simulink library "Simulation_lib"  (R2023b)
settings: Solver=VariableStepAuto  StartTime=0.0  StopTime=10.0  RelTol=1e-3
undefined symbols (not defined in the file): X, Y, Z
libraries: sm_lib x48, $bdroot x18, nesl_utility x16, fl_lib x15, ee_lib x3, simulink_extras x1
(part 1 of 3)
settings Model: Creator=FIRSTMentor  LastModifiedBy=FIRSTMentor

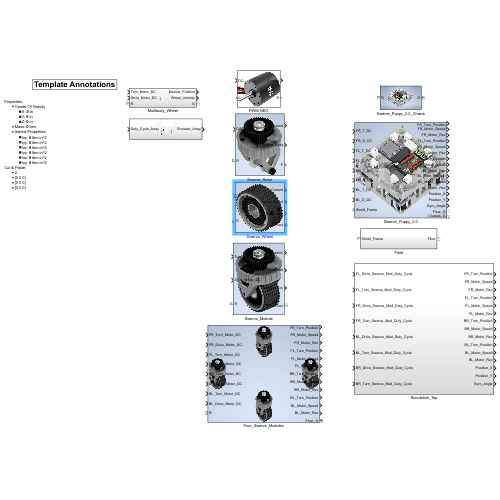
[thumbnail: Simulink's stored preview of the top-level diagram]
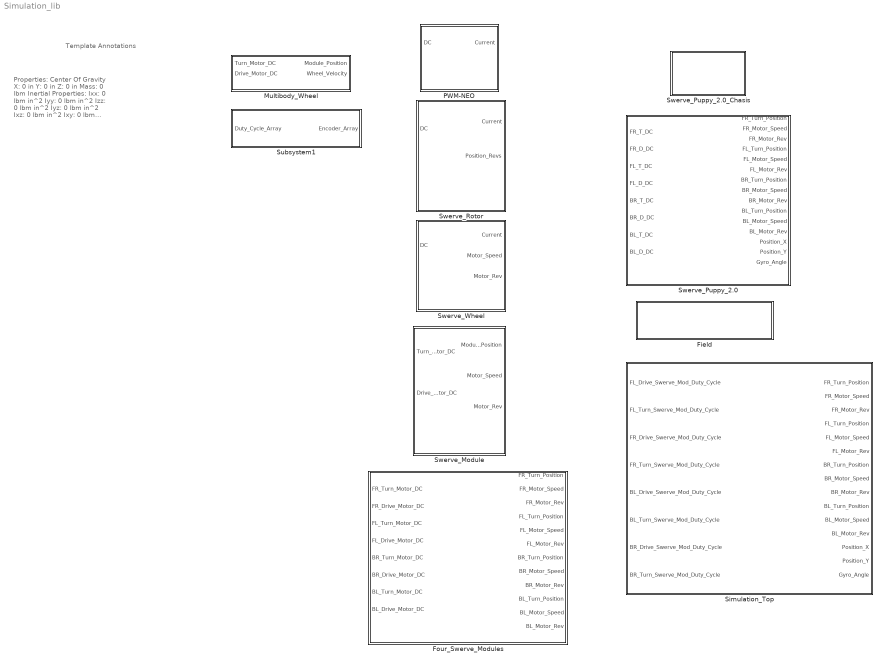
== system Simulation_lib ==
  note: Properties:
      | Center Of Gravity
      | X: 0 in
      | Y: 0 in
      | Z: 0 in
      | Mass: 0 lbm
      | Inertial Properties:
      | Ixx: 0 lbm in^2
      | Iyy: 0 lbm in^2
      | Izz: 0 lbm in^2
      | Iyz: 0 lbm in^2
      | Ixz: 0 lbm in^2
      | Ixy: 0 lbm in^2
      | Cut & Paste:
      | 0
      | [0 0 0]
      | [0 0 0]
      | [0 0 0]
  note: Template Annotations
  Field : Subsystem
  Four_Swerve_Modules : Subsystem  mask{FR_Transform=[0 0 0], FL_Transform=[0 0 0], BR_Transform=[0 0 0], BL_Transform=[0 0 0]}
      mask prompts: FR_Transform "Front Right Module Transform"; FL_Transform "Front Left Module Transform"; BR_Transform "Back Right Module Transform"; BL_Transform "Back Right Module Transform"
      mask DialogControl Instructions Prompt: Only enter the X and Y of transforms, Z should always be zero.
      mask Display: image('Four_Swerve_Modules_Icon.png'); % Use "Edit Image" on toolstrip to change.
  Multibody_Wheel : Subsystem
  PWM-NEO : Subsystem
      mask Display: image('NEO_Icon.png'); % Use "Edit Image" on toolstrip to change.
  Simulation_Top : Subsystem
  Subsystem1 : Subsystem
  Swerve_Module : Subsystem
      mask Display: image('Swerve_Wheel_Module_Icon.png'); % Use "Edit Image" on toolstrip to change.
  Swerve_Puppy_2.0 : Subsystem
      mask Display: image('Swerve_Puppy_2.0_Icon.png'); % Use "Edit Image" on toolstrip to change.
  Swerve_Puppy_2.0_Chasis : Subsystem
      mask Display: image('Swerve_Puppy_2.0_Chassis_Icon.png'); % Use "Edit Image" on toolstrip to change.
  Swerve_Rotor : Subsystem
      mask Display: image('Swerve_Rotor_Icon.png'); % Use "Edit Image" on toolstrip to change.
  Swerve_Wheel : Subsystem
      mask Display: image('Swerve_Wheel_Icon.png'); % Use "Edit Image" on toolstrip to change.

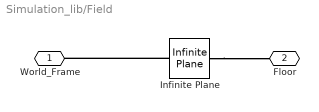
== system Simulation_lib/Field ==
  Infinite Plane : sm_lib/Curves and Surfaces/Infinite Plane  GraphicType=Rectangle  GraphicPlaneWidth=10  GraphicPlaneWidthUnits=m  GraphicPlaneHeight=10  GraphicPlaneHeightUnits=m  GraphicVisPropType=SimpleVisualProperties  GraphicDiffuseColor=[1 0.4118 0.1608]  GraphicOpacity=0.25  GraphicSpecularColor=[0.5 0.5 0.5 1.0]  GraphicAmbientColor=[0.15 0.15 0.15 1.0]  GraphicEmissiveColor=[0.0 0.0 0.0 1.0]  GraphicShininess=75
  World_Frame : PMIOPort  Side=Left
  Floor : PMIOPort  Port=2  Side=Right
  connections:
  Infinite Plane/RConn1 -- Floor/RConn1
  Infinite Plane/LConn1 -- World_Frame/RConn1

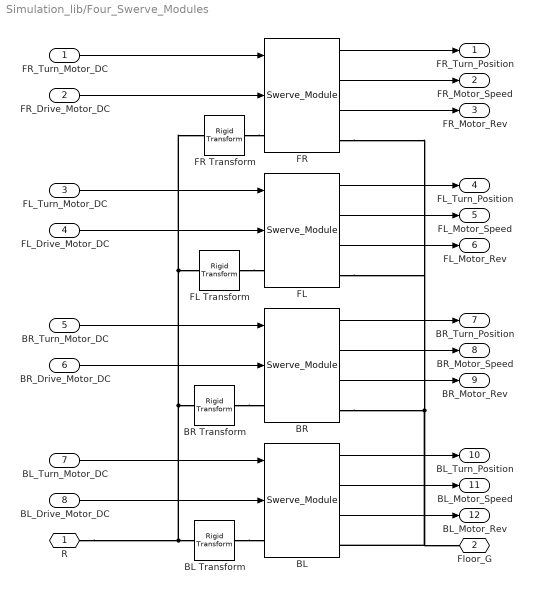
== system Simulation_lib/Four_Swerve_Modules ==
  FR_Turn_Motor_DC : Inport
  FR_Drive_Motor_DC : Inport  Port=2
  FL_Turn_Motor_DC : Inport  Port=3
  FL_Drive_Motor_DC : Inport  Port=4
  BR_Turn_Motor_DC : Inport  Port=5
  BR_Drive_Motor_DC : Inport  Port=6
  BL_Turn_Motor_DC : Inport  Port=7
  BL_Drive_Motor_DC : Inport  Port=8
  BL : $bdroot/Swerve_Module  SystemSampleTime=-1  VariantActivationTime=update diagram  AllowFlexibleInterface=on  Latency=0  AutoFrameSizeCalculation=off
  BL Transform : sm_lib/Frames and Transforms/Rigid Transform  TranslationMethod=Cartesian  TranslationStandardOffset=0  TranslationStandardOffsetUnits=m  TranslationStandardAxis=+Z  TranslationCartesianOffset=BL_Transform  TranslationCartesianOffsetUnits=in  TranslationROffset=0  TranslationROffsetUnits=m  TranslationZOffset=0  TranslationZOffsetUnits=m  TranslationThetaOffset=0  TranslationThetaOffsetUnits=deg  RotationMethod=None  RotationAngleUnits=deg  RotationStandardAxis=+Z  RotationAngle=0.0  RotationArbitraryAxis=[0 0 1]  FollAlignAxisA=+X  BaseAlignAxisA=+Y  FollAlignAxisB=+Y  BaseAlignAxisB=+Z  RotationSequenceAxes=FollowerAxes  RotationSequence=XYX  RotationSequenceAngles=[0 0 0]  RotationSequenceAnglesUnits=deg  RotationMatrix=[1 0 0; 0 1 0; 0 0 1]  Quaternion=[1 0 0 0]
  BR : $bdroot/Swerve_Module  SystemSampleTime=-1  VariantActivationTime=update diagram  AllowFlexibleInterface=on  Latency=0  AutoFrameSizeCalculation=off
  BR Transform : sm_lib/Frames and Transforms/Rigid Transform  TranslationMethod=Cartesian  TranslationStandardOffset=0  TranslationStandardOffsetUnits=m  TranslationStandardAxis=+Z  TranslationCartesianOffset=BR_Transform  TranslationCartesianOffsetUnits=in  TranslationROffset=0  TranslationROffsetUnits=m  TranslationZOffset=0  TranslationZOffsetUnits=m  TranslationThetaOffset=0  TranslationThetaOffsetUnits=deg  RotationMethod=None  RotationAngleUnits=deg  RotationStandardAxis=+Z  RotationAngle=0.0  RotationArbitraryAxis=[0 0 1]  FollAlignAxisA=+X  BaseAlignAxisA=+Y  FollAlignAxisB=+Y  BaseAlignAxisB=+Z  RotationSequenceAxes=FollowerAxes  RotationSequence=XYX  RotationSequenceAngles=[0 0 0]  RotationSequenceAnglesUnits=deg  RotationMatrix=[1 0 0; 0 1 0; 0 0 1]  Quaternion=[1 0 0 0]
  FL : $bdroot/Swerve_Module  SystemSampleTime=-1  VariantActivationTime=update diagram  AllowFlexibleInterface=on  Latency=0  AutoFrameSizeCalculation=off
  FL Transform : sm_lib/Frames and Transforms/Rigid Transform  TranslationMethod=Cartesian  TranslationStandardOffset=0  TranslationStandardOffsetUnits=m  TranslationStandardAxis=+Z  TranslationCartesianOffset=FL_Transform  TranslationCartesianOffsetUnits=in  TranslationROffset=0  TranslationROffsetUnits=m  TranslationZOffset=0  TranslationZOffsetUnits=m  TranslationThetaOffset=0  TranslationThetaOffsetUnits=deg  RotationMethod=None  RotationAngleUnits=deg  RotationStandardAxis=+Z  RotationAngle=0.0  RotationArbitraryAxis=[0 0 1]  FollAlignAxisA=+X  BaseAlignAxisA=+Y  FollAlignAxisB=+Y  BaseAlignAxisB=+Z  RotationSequenceAxes=FollowerAxes  RotationSequence=XYX  RotationSequenceAngles=[0 0 0]  RotationSequenceAnglesUnits=deg  RotationMatrix=[1 0 0; 0 1 0; 0 0 1]  Quaternion=[1 0 0 0]
  FR : $bdroot/Swerve_Module  SystemSampleTime=-1  VariantActivationTime=update diagram  AllowFlexibleInterface=on  Latency=0  AutoFrameSizeCalculation=off
  FR Transform : sm_lib/Frames and Transforms/Rigid Transform  TranslationMethod=Cartesian  TranslationStandardOffset=0  TranslationStandardOffsetUnits=m  TranslationStandardAxis=+Z  TranslationCartesianOffset=FR_Transform  TranslationCartesianOffsetUnits=in  TranslationROffset=0  TranslationROffsetUnits=m  TranslationZOffset=0  TranslationZOffsetUnits=m  TranslationThetaOffset=0  TranslationThetaOffsetUnits=deg  RotationMethod=None  RotationAngleUnits=deg  RotationStandardAxis=+Z  RotationAngle=0.0  RotationArbitraryAxis=[0 0 1]  FollAlignAxisA=+X  BaseAlignAxisA=+Y  FollAlignAxisB=+Y  BaseAlignAxisB=+Z  RotationSequenceAxes=FollowerAxes  RotationSequence=XYX  RotationSequenceAngles=[0 0 0]  RotationSequenceAnglesUnits=deg  RotationMatrix=[1 0 0; 0 1 0; 0 0 1]  Quaternion=[1 0 0 0]
  R : PMIOPort  Side=Left
  Floor_G : PMIOPort  Port=2  Side=Right
  FR_Turn_Position : Outport
  FR_Motor_Speed : Outport  Port=2
  FR_Motor_Rev : Outport  Port=3  Unit=rev
  FL_Turn_Position : Outport  Port=4
  FL_Motor_Speed : Outport  Port=5
  FL_Motor_Rev : Outport  Port=6  Unit=rev
  BR_Turn_Position : Outport  Port=7
  BR_Motor_Speed : Outport  Port=8
  BR_Motor_Rev : Outport  Port=9  Unit=rev
  BL_Turn_Position : Outport  Port=10
  BL_Motor_Speed : Outport  Port=11
  BL_Motor_Rev : Outport  Port=12  Unit=rev
  wires:
  FR_Turn_Motor_DC/1 -> FR/1
  FR_Drive_Motor_DC/1 -> FR/2
  FL_Drive_Motor_DC/1 -> FL/2
  FL_Turn_Motor_DC/1 -> FL/1
  BR_Turn_Motor_DC/1 -> BR/1
  BR_Drive_Motor_DC/1 -> BR/2
  BL_Turn_Motor_DC/1 -> BL/1
  BL_Drive_Motor_DC/1 -> BL/2
  BL/2 -> BL_Motor_Speed/1
  BL/1 -> BL_Turn_Position/1
  BR/1 -> BR_Turn_Position/1
  BR/2 -> BR_Motor_Speed/1
  FL/1 -> FL_Turn_Position/1
  FL/2 -> FL_Motor_Speed/1
  FR/1 -> FR_Turn_Position/1
  FR/2 -> FR_Motor_Speed/1
  FR/3 -> FR_Motor_Rev/1
  FL/3 -> FL_Motor_Rev/1
  BR/3 -> BR_Motor_Rev/1
  BL/3 -> BL_Motor_Rev/1
  connections:
  R/RConn1 -- FL Transform/LConn1 -- FR Transform/LConn1 -- BR Transform/LConn1 -- BL Transform/LConn1
  BL/RConn1 -- Floor_G/RConn1 -- FR/RConn1 -- FL/RConn1 -- BR/RConn1
  FR Transform/RConn1 -- FR/LConn1
  FL Transform/RConn1 -- FL/LConn1
  BR Transform/RConn1 -- BR/LConn1
  BL Transform/RConn1 -- BL/LConn1

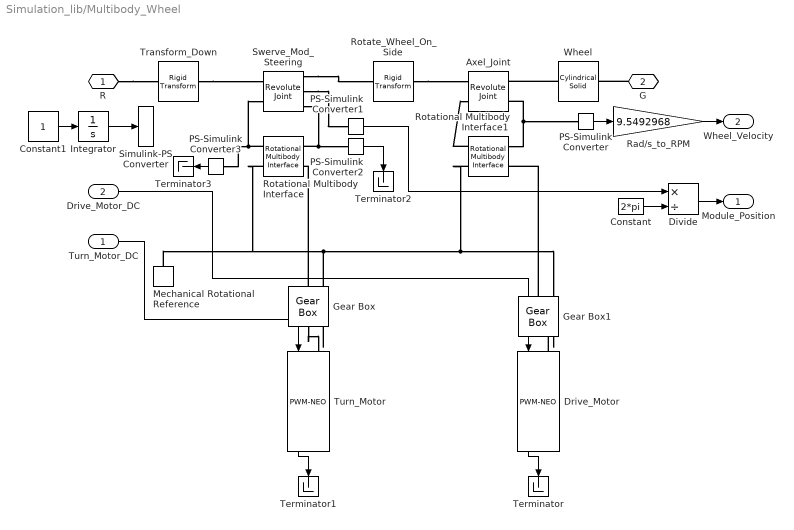
== system Simulation_lib/Multibody_Wheel ==
  Turn_Motor_DC : Inport
  Drive_Motor_DC : Inport  Port=2
  Axel_Joint : sm_lib/Joints/Revolute Joint  JointMode=Normal  SenseConstraintForce=off  SenseConstraintForceX=off  SenseConstraintForceY=off  SenseConstraintForceZ=off  SenseConstraintTorque=off  SenseConstraintTorqueX=off  SenseConstraintTorqueY=off  SenseConstraintTorqueZ=off  SenseTotalForce=off  SenseTotalForceX=off  SenseTotalForceY=off  SenseTotalForceZ=off  SenseTotalTorque=off  SenseTotalTorqueX=off  SenseTotalTorqueY=off  SenseTotalTorqueZ=off  CompositeWrenchDir=FollowerOnBase  CompositeWrenchFrame=BaseFrame  EquilibriumPosition=0  EquilibriumPositionUnits=deg  SpringStiffness=0  SpringStiffnessUnits=N*m/deg  DampingCoefficient=0  DampingCoefficientUnits=N*m/(deg/s)  TorqueActuationMode=InputTorque  MotionActuationMode=ComputedMotion  SensePosition=off  SenseVelocity=on  SenseAcceleration=off  SenseTorqueForce=off  SenseLowerLimitTorqueForce=off  SenseUpperLimitTorqueForce=off  LowerLimitSpecify=off  LowerLimitBound=-90  LowerLimitBoundUnits=deg  LowerLimitStiffness=1e4  LowerLimitStiffnessUnits=N*m/deg  LowerLimitDamping=10  LowerLimitDampingUnits=N*m/(deg/s)  LowerLimitTransitionRegionWidth=0.1  LowerLimitTransitionRegionWidthUnits=deg  UpperLimitSpecify=off  UpperLimitBound=90  UpperLimitBoundUnits=deg  UpperLimitStiffness=1e4  UpperLimitStiffnessUnits=N*m/deg  UpperLimitDamping=10  UpperLimitDampingUnits=N*m/(deg/s)  UpperLimitTransitionRegionWidth=0.1  UpperLimitTransitionRegionWidthUnits=deg  PositionTargetSpecify=off  PositionTargetPriority=High  PositionTargetValue=0  PositionTargetValueUnits=deg  VelocityTargetSpecify=off  VelocityTargetPriority=High  VelocityTargetValue=0  VelocityTargetValueUnits=deg/s
  Constant : Constant  Value=2*pi
  Constant1 : Constant
  Divide : Product  Inputs=*/
  Drive_Motor : $bdroot/PWM-NEO  SystemSampleTime=-1  VariantActivationTime=update diagram  AllowFlexibleInterface=on  Latency=0  AutoFrameSizeCalculation=off
  Gear Box : fl_lib/Mechanical/Mechanisms/Gear Box  ratio=150/7  t_in_specify=off  t_in_priority=None  t_in=0 N*m  t_in_nominal_specify=off  t_in_nominal_unit=N*m  t_in_nominal_value=1  t_out_specify=off  t_out_priority=None  t_out=0 N*m  t_out_nominal_specify=off  t_out_nominal_unit=N*m  t_out_nominal_value=1
  Gear Box1 : fl_lib/Mechanical/Mechanisms/Gear Box  ratio=8.14  t_in_specify=off  t_in_priority=None  t_in=0 N*m  t_in_nominal_specify=off  t_in_nominal_unit=N*m  t_in_nominal_value=1  t_out_specify=off  t_out_priority=None  t_out=0 N*m  t_out_nominal_specify=off  t_out_nominal_unit=N*m  t_out_nominal_value=1
  Integrator : Integrator
  Mechanical Rotational Reference : fl_lib/Mechanical/Rotational Elements/Mechanical Rotational Reference
  PS-Simulink Converter{,1..3} (4 alike) : nesl_utility/PS-Simulink Converter  PhysicalDomain=network_engine_domain  SubClassName=ps_output  LeftPortType=input  RightPortType=output  PseudoPeriodic=off  Frequencies=[]  VectorFormat=inherit  Unit=inherit  AffineConversion=off
  Rad/s_to_RPM : Gain  Gain=9.5492968
  Rotate_Wheel_On_Side : sm_lib/Frames and Transforms/Rigid Transform  TranslationMethod=None  TranslationStandardOffset=0  TranslationStandardOffsetUnits=m  TranslationStandardAxis=+Z  TranslationCartesianOffset=[0 0 0]  TranslationCartesianOffsetUnits=m  TranslationROffset=0  TranslationROffsetUnits=m  TranslationZOffset=0  TranslationZOffsetUnits=m  TranslationThetaOffset=0  TranslationThetaOffsetUnits=deg  RotationMethod=StandardAxis  RotationAngleUnits=deg  RotationStandardAxis=+X  RotationAngle=90  RotationArbitraryAxis=[0 0 1]  FollAlignAxisA=+X  BaseAlignAxisA=+Y  FollAlignAxisB=+Y  BaseAlignAxisB=+Z  RotationSequenceAxes=FollowerAxes  RotationSequence=XYX  RotationSequenceAngles=[0 0 0]  RotationSequenceAnglesUnits=deg  RotationMatrix=[1 0 0; 0 1 0; 0 0 1]  Quaternion=[1 0 0 0]
  Rotational Multibody Interface : fl_lib/Mechanical/Multibody Interfaces/Rotational Multibody Interface
  Rotational Multibody Interface1 : fl_lib/Mechanical/Multibody Interfaces/Rotational Multibody Interface
  Simulink-PS Converter : nesl_utility/Simulink-PS Converter  PhysicalDomain=network_engine_domain  SubClassName=ps_input  LeftPortType=input  RightPortType=output  PseudoPeriodic=off  Frequencies=[]  NoiseDistribution=none  NoiseParameters=[]  Unit=1  AffineConversion=on  FilteringAndDerivatives=filter  SimscapeFilterOrder=2  InputFilterTimeConstant=0.001  UdotUserProvided=2
  Swerve_Mod_Steering : sm_lib/Joints/Revolute Joint  JointMode=Normal  SenseConstraintForce=off  SenseConstraintForceX=off  SenseConstraintForceY=off  SenseConstraintForceZ=off  SenseConstraintTorque=off  SenseConstraintTorqueX=off  SenseConstraintTorqueY=off  SenseConstraintTorqueZ=off  SenseTotalForce=off  SenseTotalForceX=off  SenseTotalForceY=off  SenseTotalForceZ=off  SenseTotalTorque=off  SenseTotalTorqueX=off  SenseTotalTorqueY=off  SenseTotalTorqueZ=off  CompositeWrenchDir=FollowerOnBase  CompositeWrenchFrame=BaseFrame  EquilibriumPosition=0  EquilibriumPositionUnits=deg  SpringStiffness=0  SpringStiffnessUnits=N*m/deg  DampingCoefficient=0  DampingCoefficientUnits=N*m/(deg/s)  TorqueActuationMode=InputTorque  MotionActuationMode=ComputedMotion  SensePosition=on  SenseVelocity=on  SenseAcceleration=off  SenseTorqueForce=off  SenseLowerLimitTorqueForce=off  SenseUpperLimitTorqueForce=off  LowerLimitSpecify=off  LowerLimitBound=-90  LowerLimitBoundUnits=deg  LowerLimitStiffness=1e4  LowerLimitStiffnessUnits=N*m/deg  LowerLimitDamping=10  LowerLimitDampingUnits=N*m/(deg/s)  LowerLimitTransitionRegionWidth=0.1  LowerLimitTransitionRegionWidthUnits=deg  UpperLimitSpecify=off  UpperLimitBound=90  UpperLimitBoundUnits=deg  UpperLimitStiffness=1e4  UpperLimitStiffnessUnits=N*m/deg  UpperLimitDamping=10  UpperLimitDampingUnits=N*m/(deg/s)  UpperLimitTransitionRegionWidth=0.1  UpperLimitTransitionRegionWidthUnits=deg  PositionTargetSpecify=off  PositionTargetPriority=High  PositionTargetValue=0  PositionTargetValueUnits=deg  VelocityTargetSpecify=off  VelocityTargetPriority=High  VelocityTargetValue=0  VelocityTargetValueUnits=deg/s
  Terminator{,1..3} (4 alike) : Terminator
  Transform_Down : sm_lib/Frames and Transforms/Rigid Transform  TranslationMethod=StandardAxis  TranslationStandardOffset=-3.626112197  TranslationStandardOffsetUnits=in  TranslationStandardAxis=+Z  TranslationCartesianOffset=[0 0 0]  TranslationCartesianOffsetUnits=m  TranslationROffset=0  TranslationROffsetUnits=m  TranslationZOffset=0  TranslationZOffsetUnits=m  TranslationThetaOffset=0  TranslationThetaOffsetUnits=deg  RotationMethod=None  RotationAngleUnits=deg  RotationStandardAxis=+X  RotationAngle=90  RotationArbitraryAxis=[0 0 1]  FollAlignAxisA=+X  BaseAlignAxisA=+Y  FollAlignAxisB=+Y  BaseAlignAxisB=+Z  RotationSequenceAxes=FollowerAxes  RotationSequence=XYX  RotationSequenceAngles=[0 0 0]  RotationSequenceAnglesUnits=deg  RotationMatrix=[1 0 0; 0 1 0; 0 0 1]  Quaternion=[1 0 0 0]
  Turn_Motor : $bdroot/PWM-NEO  SystemSampleTime=-1  VariantActivationTime=update diagram  AllowFlexibleInterface=on  Latency=0  AutoFrameSizeCalculation=off
  Wheel : sm_lib/Body Elements/Cylindrical Solid  GraphicAmbientColor=[0.15 0.15 0.15 1.0]  BasedOnType=Density  CenterOfMass=[0 0 0]  CenterOfMassUnits=m  GraphicDiffuseColor=[0.5 0.5 0.5]  CylinderLength=1.645000000  CylinderLengthUnits=in  CylinderRadius=2  CylinderRadiusUnits=in  Density=1000  DensityUnits=kg/m^3  DoExposeReferenceFrame=on  GraphicEmissiveColor=[0.0 0.0 0.0 1.0]  ExportEntireGeometry=on  SerializedFrames=<Frames/>  MarkerShape=Sphere  MarkerSize=10  GraphicType=FromGeometry  InertiaType=CalculateFromGeometry  Mass=1  MassUnits=kg  MomentsOfInertia=[1 1 1]  MomentsOfInertiaUnits=kg*m^2  GraphicOpacity=1.0  ProductsOfInertia=[0 0 0]  ProductsOfInertiaUnits=kg*m^2  GraphicShininess=75  GraphicSpecularColor=[0.5 0.5 0.5 1.0]  GraphicVisPropType=SimpleVisualProperties
  R : PMIOPort  Side=Left
  G : PMIOPort  Port=2  Side=Right
  Module_Position : Outport
  Wheel_Velocity : Outport  Port=2
  wires:
  Turn_Motor_DC/1 -> Turn_Motor/1
  Drive_Motor_DC/1 -> Drive_Motor/1
  Turn_Motor/1 -> Terminator1/1
  Drive_Motor/1 -> Terminator/1
  PS-Simulink Converter/1 -> Rad/s_to_RPM/1
  Rad/s_to_RPM/1 -> Wheel_Velocity/1
  Constant/1 -> Divide/2
  Divide/1 -> Module_Position/1
  PS-Simulink Converter1/1 -> Divide/1
  Constant1/1 -> Integrator/1
  Integrator/1 -> Simulink-PS Converter/1
  PS-Simulink Converter2/1 -> Terminator2/1
  PS-Simulink Converter3/1 -> Terminator3/1
  connections:
  R/RConn1 -- Transform_Down/LConn1
  G/RConn1 -- Wheel/LConn1
  Wheel/RConn1 -- Axel_Joint/RConn1
  Rotate_Wheel_On_Side/RConn1 -- Axel_Joint/LConn1
  Rotational Multibody Interface1/LConn1 -- Axel_Joint/LConn2
  Rotational Multibody Interface/LConn2 -- Mechanical Rotational Reference/LConn1 -- Rotational Multibody Interface1/LConn2
  Gear Box1/RConn1 -- Rotational Multibody Interface1/RConn2
  Gear Box/LConn1 -- Turn_Motor/LConn1
  Rotational Multibody Interface1/RConn1 -- PS-Simulink Converter/LConn1 -- Axel_Joint/RConn2
  Swerve_Mod_Steering/RConn3 -- PS-Simulink Converter2/LConn1 -- Rotational Multibody Interface/RConn1
  Swerve_Mod_Steering/RConn2 -- PS-Simulink Converter1/LConn1
  Transform_Down/RConn1 -- Swerve_Mod_Steering/LConn1
  Swerve_Mod_Steering/RConn1 -- Rotate_Wheel_On_Side/LConn1
  Rotational Multibody Interface/LConn1 -- PS-Simulink Converter3/LConn1 -- Swerve_Mod_Steering/LConn2
  Gear Box/RConn1 -- Rotational Multibody Interface/RConn2
  Drive_Motor/LConn1 -- Gear Box1/LConn1

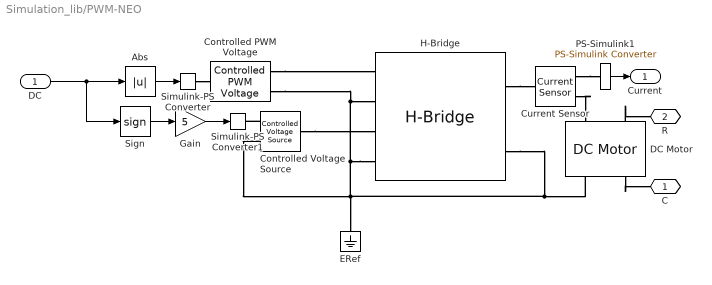
== system Simulation_lib/PWM-NEO ==
  DC : Inport
  Abs : Abs  SaturateOnIntegerOverflow=off
  Controlled PWM Voltage : ee_lib/Integrated Circuits/Controlled PWM Voltage  F=4000 Hz  TD=0 s  pulse_width_offset=0 s  pulse_min=0 s  pwm_or_av=2  event_type=1  sample_time=5e-6 s  Vmin=0 V  Vmax=5 V  Vm=5 V  u_min=0  u_max=1
      settings: InternalSimscapePortConfiguration="{\"Bottom\":[],\"Left\":[{\"id\":\"u\",\"label\":\"u\",\"type\":\"input\"}],\"Right\":[{\"id\":\"p2\",\"label\":\"PWM\",\"type\":\"foundation.electrical.electrical\"},{\"id\":\"n2\",\"label\":\"REF\",\"type\":\"foundation.electrical.electrical\"}],\"Top\":[]}"
  Controlled Voltage Source : fl_lib/Electrical/Electrical Sources/Controlled Voltage Source
  Current Sensor : fl_lib/Electrical/Electrical Sensors/Current Sensor
  DC Motor : ee_lib/Electromechanical/Brushed Motors/DC Motor  field_option=ee.enum.field_option.pm  Rf=100 Ohm  Lf=1 H  Laf=0.15 H  If0=0 A  parameterization=3  Ra=3.38 Ohm  La=0.01 H  emf_or_torque=1  Kv=0.029 V/(rad/s)  Ki=6.876e-04 N*m/A  T_stall=0.1 N*m  w_max=5700 rpm  w_rated=2910 rpm  P_rated=500 W  V_rated=12 V  lam_param=ee.enum.lam_param.current  i_noload=1.7 A  V_i_noload=12 V  J=0.0002 kg*m^2  lam=0.5e-5 N*m/(rad/s)  speed0=0 rpm  enable_fault_armature=simscape.enum.onoff.off  rev_faulted=1 / 3  G_faulted_armature=1e-5 S  fault_trigger_armature=ee.enum.faults.faultTrigger.temporal  t_fault_armature=1 s  max_permissible_current_armature=inf A  t_fail_on_current_armature=1 s  enable_fault_field=simscape.enum.onoff.off  G_faulted_field=1e-5 S  fault_trigger_field=ee.enum.faults.faultTrigger.temporal  t_fault_field=1 s  max_permissible_current_field=inf A  t_fail_on_current_field=1 s  fault_action=simscape.enum.assert.action.none  alpha=3.93e-3 1/K  Tmeas=25 degC  thermal_mass=100 J/K  initial_temperature=25 degC
  ERef : fl_lib/Electrical/Electrical Elements/Electrical Reference
  Gain : Gain  Gain=5
  H-Bridge : ee_lib/Semiconductors & Converters/Converters/H-Bridge  supply_ports=ee.enum.supply_ports.hidesupply  pwm_or_av=ee.enum.pwm_or_av.averaged  regenerative_braking_mode=ee.enum.converters.regenerative_braking_mode.always_enabled  discontinuous=ee.enum.current_profile.continuous  freewheeling_mode=1  Rload=3.38+0.1 Ohm  Lload=1e-5 H  F=4 kHz  Venable=2.5 V  Vmax=5 V  Vreverse=2.5 V  Vbrake=2.5 V  Vm=12 V  Ron=0.1 Ohm  Don=0.1 Ohm  Goff=1e-6 S  Tmeas=298.15 K  Ron2=0.1 Ohm  Don2=0.05 Ohm  Tmeas2=398.15 K  thermal_mass=100 J/K  initial_temperature=298.15 K
  PS-Simulink1 : nesl_utility/PS-Simulink Converter  PhysicalDomain=network_engine_domain  SubClassName=ps_output  LeftPortType=input  RightPortType=output  PseudoPeriodic=off  Frequencies=[]  VectorFormat=1-D array  Unit=A  AffineConversion=off
  Sign : Signum
  Simulink-PS Converter : nesl_utility/Simulink-PS Converter  PhysicalDomain=network_engine_domain  SubClassName=ps_input  LeftPortType=input  RightPortType=output  PseudoPeriodic=off  Frequencies=[]  NoiseDistribution=none  NoiseParameters=[]  Unit=1  AffineConversion=off  FilteringAndDerivatives=provide  SimscapeFilterOrder=1  InputFilterTimeConstant=0.001  UdotUserProvided=0
  Simulink-PS Converter1 : nesl_utility/Simulink-PS Converter  PhysicalDomain=network_engine_domain  SubClassName=ps_input  LeftPortType=input  RightPortType=output  PseudoPeriodic=off  Frequencies=[]  NoiseDistribution=none  NoiseParameters=[]  Unit=1  AffineConversion=off  FilteringAndDerivatives=zero  SimscapeFilterOrder=1  InputFilterTimeConstant=0.001  UdotUserProvided=0
  C : PMIOPort  Side=Left
  R : PMIOPort  Port=2  Side=Right
  Current : Outport
  wires:
  PS-Simulink1/1 -> Current/1
  Abs/1 -> Simulink-PS Converter/1
  DC/1 -> Sign/1, Abs/1
  Sign/1 -> Gain/1
  Gain/1 -> Simulink-PS Converter1/1
  connections:
  Current Sensor/RConn1 -- PS-Simulink1/LConn1
  H-Bridge/RConn1 -- Current Sensor/LConn1
  Simulink-PS Converter/RConn1 -- Controlled PWM Voltage/LConn1
  DC Motor/RConn2 -- C/RConn1
  DC Motor/LConn2 -- R/RConn1
  Current Sensor/RConn2 -- DC Motor/LConn1
  H-Bridge/LConn4 -- Controlled PWM Voltage/RConn2 -- H-Bridge/LConn2 -- Controlled Voltage Source/RConn2 -- ERef/LConn1 -- H-Bridge/RConn2 -- DC Motor/RConn1
  Controlled Voltage Source/LConn1 -- H-Bridge/LConn3
  Controlled Voltage Source/RConn1 -- Simulink-PS Converter1/RConn1
  Controlled PWM Voltage/RConn1 -- H-Bridge/LConn1

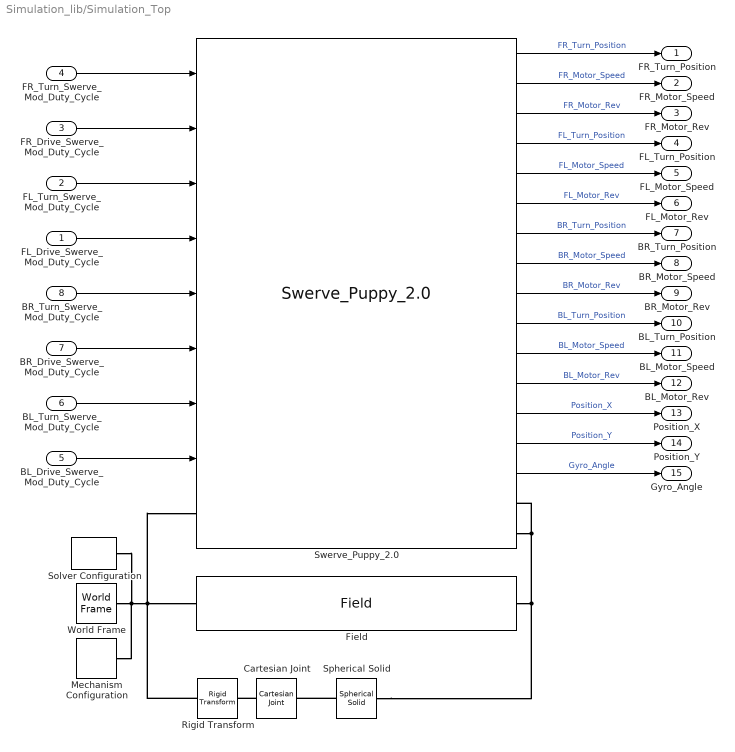
== system Simulation_lib/Simulation_Top ==
  FL_Drive_Swerve_Mod_Duty_Cycle : Inport
  FL_Turn_Swerve_Mod_Duty_Cycle : Inport  Port=2
  FR_Drive_Swerve_Mod_Duty_Cycle : Inport  Port=3
  FR_Turn_Swerve_Mod_Duty_Cycle : Inport  Port=4
  BL_Drive_Swerve_Mod_Duty_Cycle : Inport  Port=5
  BL_Turn_Swerve_Mod_Duty_Cycle : Inport  Port=6
  BR_Drive_Swerve_Mod_Duty_Cycle : Inport  Port=7
  BR_Turn_Swerve_Mod_Duty_Cycle : Inport  Port=8
  Cartesian Joint : sm_lib/Joints/Cartesian Joint  JointMode=Normal  SenseConstraintForce=off  SenseConstraintForceX=off  SenseConstraintForceY=off  SenseConstraintForceZ=off  SenseConstraintTorque=off  SenseConstraintTorqueX=off  SenseConstraintTorqueY=off  SenseConstraintTorqueZ=off  SenseTotalForce=off  SenseTotalForceX=off  SenseTotalForceY=off  SenseTotalForceZ=off  SenseTotalTorque=off  SenseTotalTorqueX=off  SenseTotalTorqueY=off  SenseTotalTorqueZ=off  CompositeWrenchDir=FollowerOnBase  CompositeWrenchFrame=BaseFrame  PxEquilibriumPosition=0  PxEquilibriumPositionUnits=m  PxSpringStiffness=0  PxSpringStiffnessUnits=N/m  PxDampingCoefficient=0  PxDampingCoefficientUnits=N/(m/s)  PxTorqueActuationMode=NoTorque  PxMotionActuationMode=ComputedMotion  PxSensePosition=off  PxSenseVelocity=off  PxSenseAcceleration=off  PxSenseTorqueForce=off  PxSenseLowerLimitTorqueForce=off  PxSenseUpperLimitTorqueForce=off  PxLowerLimitSpecify=off  PxLowerLimitBound=-1  PxLowerLimitBoundUnits=m  PxLowerLimitStiffness=1e6  PxLowerLimitStiffnessUnits=N/m  PxLowerLimitDamping=1e3  PxLowerLimitDampingUnits=N/(m/s)  PxLowerLimitTransitionRegionWidth=1e-4  PxLowerLimitTransitionRegionWidthUnits=m  PxUpperLimitSpecify=off  PxUpperLimitBound=1  PxUpperLimitBoundUnits=m  PxUpperLimitStiffness=1e6  PxUpperLimitStiffnessUnits=N/m  PxUpperLimitDamping=1e3  PxUpperLimitDampingUnits=N/(m/s)  PxUpperLimitTransitionRegionWidth=1e-4  PxUpperLimitTransitionRegionWidthUnits=m  PxPositionTargetSpecify=off  PxPositionTargetPriority=High  PxPositionTargetValue=0  PxPositionTargetValueUnits=m  PxVelocityTargetSpecify=off  PxVelocityTargetPriority=High  PxVelocityTargetValue=0  PxVelocityTargetValueUnits=m/s  PyEquilibriumPosition=0  PyEquilibriumPositionUnits=m  PySpringStiffness=0  PySpringStiffnessUnits=N/m  PyDampingCoefficient=0  PyDampingCoefficientUnits=N/(m/s)  PyTorqueActuationMode=NoTorque  PyMotionActuationMode=ComputedMotion  PySensePosition=off  PySenseVelocity=off  PySenseAcceleration=off  PySenseTorqueForce=off  PySenseLowerLimitTorqueForce=off  PySenseUpperLimitTorqueForce=off  PyLowerLimitSpecify=off  PyLowerLimitBound=-1  PyLowerLimitBoundUnits=m  PyLowerLimitStiffness=1e6  PyLowerLimitStiffnessUnits=N/m  PyLowerLimitDamping=1e3  PyLowerLimitDampingUnits=N/(m/s)  PyLowerLimitTransitionRegionWidth=1e-4  PyLowerLimitTransitionRegionWidthUnits=m  PyUpperLimitSpecify=off  PyUpperLimitBound=1  PyUpperLimitBoundUnits=m  PyUpperLimitStiffness=1e6  PyUpperLimitStiffnessUnits=N/m  PyUpperLimitDamping=1e3  PyUpperLimitDampingUnits=N/(m/s)  PyUpperLimitTransitionRegionWidth=1e-4  PyUpperLimitTransitionRegionWidthUnits=m  PyPositionTargetSpecify=off  PyPositionTargetPriority=High  PyPositionTargetValue=0  PyPositionTargetValueUnits=m  PyVelocityTargetSpecify=off  PyVelocityTargetPriority=High  PyVelocityTargetValue=0  PyVelocityTargetValueUnits=m/s  PzEquilibriumPosition=0  PzEquilibriumPositionUnits=m  PzSpringStiffness=0  PzSpringStiffnessUnits=N/m  PzDampingCoefficient=0  PzDampingCoefficientUnits=N/(m/s)  PzTorqueActuationMode=NoTorque  PzMotionActuationMode=ComputedMotion  PzSensePosition=off  PzSenseVelocity=off  PzSenseAcceleration=off  PzSenseTorqueForce=off  PzSenseLowerLimitTorqueForce=off  PzSenseUpperLimitTorqueForce=off  PzLowerLimitSpecify=off  PzLowerLimitBound=-1  PzLowerLimitBoundUnits=m  PzLowerLimitStiffness=1e6  PzLowerLimitStiffnessUnits=N/m  PzLowerLimitDamping=1e3  PzLowerLimitDampingUnits=N/(m/s)  PzLowerLimitTransitionRegionWidth=1e-4  PzLowerLimitTransitionRegionWidthUnits=m  PzUpperLimitSpecify=off  PzUpperLimitBound=1  PzUpperLimitBoundUnits=m  PzUpperLimitStiffness=1e6  PzUpperLimitStiffnessUnits=N/m  PzUpperLimitDamping=1e3  PzUpperLimitDampingUnits=N/(m/s)  PzUpperLimitTransitionRegionWidth=1e-4  PzUpperLimitTransitionRegionWidthUnits=m  PzPositionTargetSpecify=off  PzPositionTargetPriority=High  PzPositionTargetValue=0  PzPositionTargetValueUnits=m  PzVelocityTargetSpecify=off  PzVelocityTargetPriority=High  PzVelocityTargetValue=0  PzVelocityTargetValueUnits=m/s
  Field : $bdroot/Field  SystemSampleTime=-1  VariantActivationTime=update diagram  AllowFlexibleInterface=on  Latency=0  AutoFrameSizeCalculation=off
  Mechanism Configuration : sm_lib/Utilities/Mechanism Configuration  UniformGravity=Constant  GravityVector=[0 0 -9.80665]  GravityVectorUnits=m/s^2  LinearizationDelta=0.001  JointModeTransitionNonlinearIterations=2
  Rigid Transform : sm_lib/Frames and Transforms/Rigid Transform  TranslationMethod=StandardAxis  TranslationStandardOffset=1  TranslationStandardOffsetUnits=m  TranslationStandardAxis=+Z  TranslationCartesianOffset=[0 0 0]  TranslationCartesianOffsetUnits=m  TranslationROffset=0  TranslationROffsetUnits=m  TranslationZOffset=0  TranslationZOffsetUnits=m  TranslationThetaOffset=0  TranslationThetaOffsetUnits=deg  RotationMethod=None  RotationAngleUnits=deg  RotationStandardAxis=+Z  RotationAngle=2  RotationArbitraryAxis=[0 0 1]  FollAlignAxisA=+X  BaseAlignAxisA=+Y  FollAlignAxisB=+Y  BaseAlignAxisB=+Z  RotationSequenceAxes=FollowerAxes  RotationSequence=XYX  RotationSequenceAngles=[0 0 0]  RotationSequenceAnglesUnits=deg  RotationMatrix=[1 0 0; 0 1 0; 0 0 1]  Quaternion=[1 0 0 0]
  Solver Configuration : nesl_utility/Solver Configuration  PhysicalDomain=network_engine_domain  SubClassName=solver  LeftPortType=input  RightPortType=generic  Tones=[]  Harmonics=[]  SimulateNoise=off  Profile=off  UseLocalSampling=off  EnableSwitchedLinearOptims=on  FrequencyDomain=off  UseCCode=off  RelTol=0.001  AbsTol=0.001  MinStep=1e-09  ToWorkspace=off  RevertToSquareIcSolve=off  NumHomotopyIterations=100  PhasorMode=off  PhasorModeNumHarmonics=1  ConsistencySolver=NEWTON_XTOL_AFTER_FTOL  IndexReductionMethod=DerivativeReplacement  DoDC=off  ResidualTolerance=1e-09  ConsistencyTolSource=GLOBAL  ConsistencyAbsTol=0.001  ConsistencyRelTol=0.001  ConsistencyTolFactor=0.001  UseLocalSolver=off  LocalSolverChoice=NE_BACKWARD_EULER_ADVANCER  ResolveIndetEquations=on  FunctionEvalNumThread=1  LocalSolverSampleTime=0.001  DoFixedCost=off  MaxNonlinIter=3  MaxModeIter=2  ComputeImpulses=off  ImpulseIterations=2  LinearAlgebra=auto  LinearAlgebraNumThread=0  EquationFormulation=NE_TIME_EF  DelaysMemoryBudget=1024  AutomaticFiltering=on  FilteringTimeConstant=0.001  PartitionStorageMethod=AS_NEEDED  PartitionMemoryBudget=1024  PartitionMethod=ROBUST  MultibodyUseLocalSolver=off  MultibodyLocalSolverChoice=ODE1  MultibodyLocalSolverSampleTime=0.001
  Spherical Solid : sm_lib/Body Elements/Spherical Solid  GraphicAmbientColor=[0.15 0.15 0.15 1.0]  BasedOnType=Density  CenterOfMass=[0 0 0]  CenterOfMassUnits=m  GraphicDiffuseColor=[0.5 0.5 0.5]  Density=1000  DensityUnits=kg/m^3  DoExposeReferenceFrame=on  GraphicEmissiveColor=[0.0 0.0 0.0 1.0]  ExportEntireGeometry=on  SerializedExposedGeometries=<exposedGeometries><exposedGeom><rawGeomId>entire</rawGeomId><exposedGeomId>G</exposedGeomId></exposedGeom></exposedGeometries>  SerializedFrames=<Frames/>  MarkerShape=Sphere  MarkerSize=10  GraphicType=FromGeometry  InertiaType=CalculateFromGeometry  Mass=1  MassUnits=kg  MomentsOfInertia=[1 1 1]  MomentsOfInertiaUnits=kg*m^2  GraphicOpacity=1.0  ProductsOfInertia=[0 0 0]  ProductsOfInertiaUnits=kg*m^2  GraphicShininess=75  GraphicSpecularColor=[0.5 0.5 0.5 1.0]  SphereRadius=0.3556/2  SphereRadiusUnits=m  GraphicVisPropType=SimpleVisualProperties
  Swerve_Puppy_2.0 : $bdroot/Swerve_Puppy_2.0  SystemSampleTime=-1  VariantActivationTime=update diagram  AllowFlexibleInterface=on  Latency=0  AutoFrameSizeCalculation=off
  World Frame : sm_lib/Frames and Transforms/World Frame
  FR_Turn_Position : Outport
  FR_Motor_Speed : Outport  Port=2
  FR_Motor_Rev : Outport  Port=3
  FL_Turn_Position : Outport  Port=4
  FL_Motor_Speed : Outport  Port=5
  FL_Motor_Rev : Outport  Port=6
  BR_Turn_Position : Outport  Port=7
  BR_Motor_Speed : Outport  Port=8
  BR_Motor_Rev : Outport  Port=9
  BL_Turn_Position : Outport  Port=10
  BL_Motor_Speed : Outport  Port=11
  BL_Motor_Rev : Outport  Port=12
  Position_X : Outport  Port=13
  Position_Y : Outport  Port=14
  Gyro_Angle : Outport  Port=15
  wires:
  FR_Turn_Swerve_Mod_Duty_Cycle/1 -> Swerve_Puppy_2.0/1
  FR_Drive_Swerve_Mod_Duty_Cycle/1 -> Swerve_Puppy_2.0/2
  FL_Turn_Swerve_Mod_Duty_Cycle/1 -> Swerve_Puppy_2.0/3
  FL_Drive_Swerve_Mod_Duty_Cycle/1 -> Swerve_Puppy_2.0/4
  BR_Turn_Swerve_Mod_Duty_Cycle/1 -> Swerve_Puppy_2.0/5
  BR_Drive_Swerve_Mod_Duty_Cycle/1 -> Swerve_Puppy_2.0/6
  BL_Turn_Swerve_Mod_Duty_Cycle/1 -> Swerve_Puppy_2.0/7
  BL_Drive_Swerve_Mod_Duty_Cycle/1 -> Swerve_Puppy_2.0/8
  Swerve_Puppy_2.0/15 -> Gyro_Angle/1  "Gyro_Angle"
  Swerve_Puppy_2.0/1 -> FR_Turn_Position/1  "FR_Turn_Position"
  Swerve_Puppy_2.0/2 -> FR_Motor_Speed/1  "FR_Motor_Speed"
  Swerve_Puppy_2.0/4 -> FL_Turn_Position/1  "FL_Turn_Position"
  Swerve_Puppy_2.0/5 -> FL_Motor_Speed/1  "FL_Motor_Speed"
  Swerve_Puppy_2.0/7 -> BR_Turn_Position/1  "BR_Turn_Position"
  Swerve_Puppy_2.0/8 -> BR_Motor_Speed/1  "BR_Motor_Speed"
  Swerve_Puppy_2.0/10 -> BL_Turn_Position/1  "BL_Turn_Position"
  Swerve_Puppy_2.0/11 -> BL_Motor_Speed/1  "BL_Motor_Speed"
  Swerve_Puppy_2.0/3 -> FR_Motor_Rev/1  "FR_Motor_Rev"
  Swerve_Puppy_2.0/6 -> FL_Motor_Rev/1  "FL_Motor_Rev"
  Swerve_Puppy_2.0/9 -> BR_Motor_Rev/1  "BR_Motor_Rev"
  Swerve_Puppy_2.0/12 -> BL_Motor_Rev/1  "BL_Motor_Rev"
  Swerve_Puppy_2.0/13 -> Position_X/1  "Position_X"
  Swerve_Puppy_2.0/14 -> Position_Y/1  "Position_Y"
  connections:
  World Frame/RConn1 -- Mechanism Configuration/RConn1 -- Solver Configuration/RConn1 -- Rigid Transform/LConn1 -- Swerve_Puppy_2.0/LConn1 -- Field/LConn1
  Field/RConn1 -- Swerve_Puppy_2.0/RConn2 -- Swerve_Puppy_2.0/RConn1 -- Spherical Solid/LConn1
  Spherical Solid/RConn1 -- Cartesian Joint/RConn1
  Cartesian Joint/LConn1 -- Rigid Transform/RConn1
